simulink model "modelo_f_HIL"  (R2024b)
settings: Solver=ode15s  StartTime=0.0  StopTime=inf  FixedStep=T_s  RelTol=1e-3
InitFcn:
  | clc
  | clear
  | close all
  | clear all
  | clear mex
  | parametros
  | gain_CL
  | calculo_observador_carro
  | calculo_observador_izaje
values from neighbouring files (symbols this model uses):
  b_cx = 1e6    (= 1000000)    [parametros.m]
  b_cy = 1e7    (= 10000000)    [parametros.m]
  b_hb = 1e8    (= 100000000)    [parametros.m]
  b_hd = 8    [parametros.m]
  b_hm = 18    [parametros.m]
  b_t = 90    [parametros.m]
  b_tb = 5e6    (= 5000000)    [parametros.m]
  b_td = 1.8    [parametros.m]
  b_tm = 6    [parametros.m]
  b_tw = 3e3    (= 3000)    [parametros.m]
  b_wu = 150    [parametros.m]
  container_pillars = container_pillars(randperm(19))    [parametros.m]
  escenario = 1    [parametros.m]
  g = 9.80665    [parametros.m]
  H_c = 2.59    [parametros.m]
  H_truck = 1    [parametros.m]
  i_h = 22    [parametros.m]
  i_t = 30    [parametros.m]
  J_hd_hEb = 3800    [parametros.m]
  J_hm_hb = 30    [parametros.m]
  J_td = 1200    [parametros.m]
  J_tm_tb = 7    [parametros.m]
  K_cy = 1.8e9    (= 1800000000)    [parametros.m]
  K_tw = 4.8e5    (= 480000)    [parametros.m]
  k_wu = 2.36e8    (= 236000000)    [parametros.m]
  l_h0 = (Y_t0-y_l0)    (= 15)    [parametros.m]
  l_h_max = Y_t0-y_h_min    (= 65)    [parametros.m]
  l_h_maxE = l_h_max+0.5    (= 65.5)    [parametros.m]
  l_h_min = Y_t0-y_h_max    (= 5)    [parametros.m]
  l_h_minE = l_h_min-0.5    (= 4.5)    [parametros.m]
  M_cmax = 50000    [parametros.m]
  M_cmin = 2000    [parametros.m]
  M_s = 15000    [parametros.m]
  M_t = 30000    [parametros.m]
  r_hd = 0.75    [parametros.m]
  r_td = 0.50    (= 0.5)    [parametros.m]
  T_hbMax = 5e4    (= 50000)    [parametros.m]
  T_hEbMax = 1.1e6    (= 1100000)    [parametros.m]
  T_hmMax = 2e4    (= 20000)    [parametros.m]
  T_s = 0.001    [parametros.m]
  T_s0 = 0.001    [parametros.m]
  T_s1 = 0.020    (= 0.02)    [parametros.m]
  T_s2 = 0.020    (= 0.02)    [parametros.m]
  T_tbMax = 5e3    (= 5000)    [parametros.m]
  T_tmMax = 4e3    (= 4000)    [parametros.m]
  tau_tm = 1e-3    (= 0.001)    [parametros.m]
  theta_hm0 = -l_h0*i_h*2/r_hd    (= -880)    [parametros.m]
  theta_tm0 = (x_t0)*i_t/r_td    (= -1500)    [parametros.m]
  trucks0 = [0, 0, 0, 0, 0]    [parametros.m]
  v_h_max_load = 1.5    [parametros.m]
  v_h_max_noload = 3    [parametros.m]
  v_lx0 = 0    [parametros.m]
  v_ly0 = 0    [parametros.m]
  v_t0 = 0    [parametros.m]
  v_t_max = 4    [parametros.m]
  W_c = ctrb(A, B_c(:,1))    [CyO_carro.m]    (also in CyO_izaje.m; parametros.m = 2.44)
  w_hm0 = 0    [parametros.m]
  w_hm_rated = v_h_max_load*2*i_h/r_hd    (= 88)    [parametros.m]
  w_tm0 = (v_t0)*i_t/r_td    (= 0)    [parametros.m]
  x_c0_left = -35    [parametros.m]
  x_c0_right = 55    [parametros.m]
  x_containers_left_lim = 1.5    [parametros.m]
  x_containers_right_lim = 48.5    [parametros.m]
  x_l0 = x_t0    (= -25)    [parametros.m]
  x_lidar_offset = 3.0    (= 3)    [parametros.m]
  x_t0 = -25    [parametros.m]
  x_t_max = 50    [parametros.m]
  x_t_maxE = x_t_max+0.5    (= 50.5)    [parametros.m]
  x_t_min = -30    [parametros.m]
  x_t_minE = x_t_min-0.5    (= -30.5)    [parametros.m]
  y_h_min = -20    [parametros.m]
  y_l0 = 30    [parametros.m]
  Y_sb = 5.0    (= 5)    [parametros.m]
  Y_t0 = 45    [parametros.m]
libraries: opcualib x2, dspnetwork x2, dspsigops x1, simulink x1
(part 3 of 3)

== matlab function modelo_f_HIL/UDP: Controller reader/MATLAB Function ==
  data: trolley_cmd output; hoist_cmd output; system_on output; auto_mode output; twistlock output; sway_ctrl output; emergency output; emgy_ack output; data input
function [trolley_cmd, hoist_cmd, system_on, auto_mode, twistlock, sway_ctrl, emergency, emgy_ack] = parse_udp_packet(data)
% parse_udp_packet  Desempaqueta el datagrama de 14 bytes enviado por controller_reader.py
%
% Entrada:
%   data  : uint8(1x14) — bytes crudos del bloque UDP Receive
%
% Salidas (todas double):
%   trolley_cmd  [-4.0 .. +4.0] m/s   consigna velocidad carro
%   hoist_cmd    [-1.5 .. +1.5] m/s   consigna velocidad izaje
%   system_on    0/1   Sistema ON/OFF
%   auto_mode    0/1   Modo automático activo
%   twistlock    0/1   0=Abierto 1=Cerrado
%   sway_ctrl    0/1   Control de balanceo ON/OFF
%   emergency    0/1   Emergencia activa
%   emgy_ack     0/1   ACK de emergencia global
%
% Formato del paquete Python: struct.pack('!ffBBBBBB', ...)
%   Big-endian: bytes 1-4 float32, 5-8 float32, 9-14 uint8
% -----------------------------------------------------------------------

% Valores por defecto (paquete malformado o vacío)
trolley_cmd = 0;
hoist_cmd   = 0;
system_on   = 0;
auto_mode   = 0;
twistlock   = 0;
sway_ctrl   = 0;
emergency   = 0;
emgy_ack    = 0;

if numel(data) < 14
    return
end

raw = uint8(data(:)');   % forzar fila 1x14

% ── Floats big-endian → invertir bytes antes de typecast ──────────────
%    Python '!' = big-endian; x86/MATLAB = little-endian
trolley_cmd = double(typecast(raw(4:-1:1), 'single'));
hoist_cmd   = double(typecast(raw(8:-1:5), 'single'));

% ── Flags uint8 (un byte cada uno) ────────────────────────────────────
system_on = double(raw(9));
auto_mode = double(raw(10));
twistlock = double(raw(11));
sway_ctrl = double(raw(12));
emergency = double(raw(13));
emgy_ack  = double(raw(14));

== matlab function modelo_f_HIL/Nivel 2/MATLAB Function5 ==
  data: x_t_ref input; v_t_ref output; x_hat input; v_t_ff input; v_td_hat input; v_max input
function v_t_ref = controlador_posicion(x_t_ref, x_hat, v_t_ff,v_td_hat, v_max)

    % Kp = 2;
    Kd = 0;
    Kp = .11;

    e_x = x_t_ref - x_hat;
    % e_v = v_t_ff - v_td_hat;

    % v_calculada = (Kp * e_x) + e_v* Kd;
    v_calculada = Kp * e_x  + v_t_ff* Kd;

    if v_calculada > v_max
        v_t_ref = v_max;
    elseif v_calculada < -v_max
        v_t_ref = -v_max;
    else
        v_t_ref = v_calculada;
    end
end

== matlab function modelo_f_HIL/Nivel 2/MATLAB Function6 ==
  data: dl_h_ref output; l_h_ref input; l_h_sensor input; dl_h_ff input; m_est input
function dl_h_ref = controlador_posicion(l_h_ref, l_h_sensor, dl_h_ff, m_est)

    Kp = 0.5;

    e_l_h = l_h_ref - l_h_sensor;

    dl_h_ref = Kp * e_l_h; %+ dl_h_ff;

    if m_est > 16000
        dl_h_ref = min([1.5, max([dl_h_ref, -1.5])]);
    else
        dl_h_ref = min([3, max([dl_h_ref, -3])]);
    end
end

== matlab function modelo_f_HIL/Nivel 2/MATLAB Function2 ==
  data: sway_ctr_gain input; theta_hm input; theta_l input; v_balanceo output; w_l input; w_hm_hat input; enable input
function v_balanceo = controlador_balanceo_torque(sway_ctr_gain, theta_hm, theta_l, w_l, w_hm_hat, enable)
    persistent g r_hd i_h DEG2RAD 

    if isempty(g)
        DEG2RAD = pi/180;
        g       = 9.8066;
        r_hd    = 0.75;
        i_h     = 22;
    end

    if ~enable
        v_balanceo = 0;
        return;
    end

    l      = theta_hm * (-r_hd)/(i_h*2);
    dl_dt  = w_hm_hat * (-r_hd)/(i_h*2);
    l_seg  = max(l, 0.1);
    th_sat = max(-80*DEG2RAD, min(80*DEG2RAD, theta_l));
    w_o    = sqrt(g / l_seg);
    K_do   = (2*w_o*l_seg - 2*dl_dt) / cos(th_sat);
    v_balanceo = K_do * theta_l;   

end

== matlab function modelo_f_HIL/Nivel 2/Subsistema físico/MATLAB Function ==
  data: x_c0_left input; y_c0_contacto output; x_c0_right input; Y_sb input; W_c input; y_h_min input; H_c input; x_lidar_offset input; x_l input; container_pillars input; TLK input; x_t input; trucks0 input; H_truck input; Ts input; rand_in input; escenario input; x_containers_left_lim input; x_containers_right_lim input; t_camion_transicion input; y_c0_lidar output; containers_pillars_state output size=1,19; trucks_state output; trucks_has_load output; carga_tomada output
function [y_c0_contacto, y_c0_lidar, containers_pillars_state, trucks_state, trucks_has_load, carga_tomada] = ...
    perfil_suelo(x_c0_left, x_c0_right, Y_sb, W_c, y_h_min, H_c, x_lidar_offset, x_l, ...
                 container_pillars, TLK, x_t, trucks0, H_truck, Ts, rand_in, escenario, ...
                 x_containers_left_lim, x_containers_right_lim, t_camion_transicion)

persistent n_containers x_grid2 tlk_prev dx_grid idx_posiciones
persistent trucks_state_p trucks_has_load_p idx_trucks lambda_truck grupo_camion
persistent idx_zona_min idx_zona_max
persistent truck_en_transicion truck_timer
persistent carga_tomada_p

% Declarar tamaño variable seguro para arreglos dinámicos persistentes
coder.varsize('x_grid2', [1, 10000], [false, true]);
coder.varsize('n_containers', [1, 10000], [false, true]);

%% Inicialización de perfil de contenedores
if isempty(n_containers)
    dx_grid = 0.01;
    x_grid2 = x_c0_left : dx_grid : x_c0_right;
    n_containers = zeros(1, length(x_grid2));
    tlk_prev     = false;
    
    % --- Limites de la zona valida de contenedores (nunca escribir fuera de esto) ---
    idx_zona_min = round((x_containers_left_lim - x_c0_left) / dx_grid) + 1;
    idx_zona_max = round((x_containers_right_lim - x_c0_left) / dx_grid) + 1;
    idx_zona_min = max(1, min(length(x_grid2), idx_zona_min));
    idx_zona_max = max(1, min(length(x_grid2), idx_zona_max));
    
    % --- Carga inicial de pilas (19 posiciones estáticas garantizadas 1x19) ---
    n_pilares = 19;
    x_posiciones = linspace(x_containers_left_lim, x_containers_right_lim, n_pilares);
    idx_posiciones = zeros(1, 19);
    medio_ancho_idx = round((W_c/2) / dx_grid);
    
    for k = 1:n_pilares
        idx_pos = round((x_posiciones(k) - x_c0_left) / dx_grid) + 1;
        idx_pos = max(1, min(length(x_grid2), idx_pos));
        idx_posiciones(k) = idx_pos;
        
        idx_ini = max([1, idx_pos - medio_ancho_idx, idx_zona_min]);
        idx_fin = min([length(x_grid2), idx_pos + medio_ancho_idx, idx_zona_max]);
        n_containers(idx_ini:idx_fin) = container_pillars(k);
    end
    
    % --- Inicialización de camiones ---
    x_trucks_left = [-25 -20 -15 -10 -5];
    idx_trucks = zeros(1, 5);
    for k = 1:5
        idx_t = round((x_trucks_left(k) - x_c0_left) / dx_grid) + 1;
        idx_trucks(k) = max(1, min(length(x_grid2), idx_t));
    end
    
    trucks_state_p      = double(trucks0(:)'); % Forzar dimensiones 1x5
    trucks_has_load_p   = zeros(1,5);
    lambda_truck        = -log(0.5) / 60;
    grupo_camion        = ones(1,5);
    truck_en_transicion = zeros(1,5);
    truck_timer         = zeros(1,5);
    carga_tomada_p      = false;
end

%% Índice más cercano a x_l (posición de la carga)
idx = round((x_l - x_c0_left) / dx_grid) + 1;
idx = max(1, min(length(x_grid2), idx));
medio_ancho_idx = round((W_c/2) / dx_grid);

% La ventana de escritura/lectura de la carga nunca invade fuera
% de la zona valida de contenedores (evita que se mezcle con Y_sb u otras zonas)
idx_ini_l = max([1, idx - medio_ancho_idx, idx_zona_min]);
idx_fin_l = min([length(x_grid2), idx + medio_ancho_idx, idx_zona_max]);

%% Flancos de TLK
tlk_bool      = logical(TLK);
flanco_bajada = tlk_prev && ~tlk_bool;   % Soltar carga (1 -> 0)
flanco_subida = ~tlk_prev && tlk_bool;   % Tomar carga (0 -> 1)
tlk_prev      = tlk_bool;

% carga_tomada refleja directamente si el spreader esta enganchado a algo
% (TLK activo).
if flanco_subida
    carga_tomada_p = true;
elseif flanco_bajada
    carga_tomada_p = false;
end
carga_tomada = carga_tomada_p;

%% Identificar si la carga está sobre la posición de un camión
W_trucks_idx = round((W_c/2) / dx_grid);
sobre_camion_k = 0;
for k = 1:5
    if abs(idx - idx_trucks(k)) <= W_trucks_idx && trucks_state_p(k) == 1
        sobre_camion_k = k;
        break;
    end
end

%% Manejo de escenarios
if escenario ~= 0
    switch escenario
        case 1
            grupo_camion = ones(1,5);     % Carga
        case 2
            grupo_camion = 2*ones(1,5);   % Descarga
        case 3
            grupo_camion = [2 2 1 1 1];   % Mixto
    end
end

if sobre_camion_k > 0 && escenario ~= 0
    k = sobre_camion_k;
    if flanco_subida && grupo_camion(k) == 1 && trucks_has_load_p(k) == 1
        % El camión libera la carga instantáneamente al spreader
        trucks_has_load_p(k) = 0; 
        
        % Se arma un timer. El camión VACÍO se retira recién después
        truck_en_transicion(k) = 1;
        truck_timer(k) = 0;
        
    elseif flanco_bajada && grupo_camion(k) == 2 && trucks_has_load_p(k) == 0
        % NUEVA CORRECCIÓN: Al depositar, el camión recibe la carga instantáneamente
        trucks_has_load_p(k) = 1; 
        
        % Inicia el timer. El camión (CON CARGA) se retirará después de t_camion_transicion
        truck_en_transicion(k) = 1;
        truck_timer(k) = 0;
    end
else
    % Solo modifica n_containers si la ventana de escritura cae dentro de la zona valida
    if idx_fin_l >= idx_ini_l
        
        % Buscar el pilar fijo más cercano a la posición de la carga
        [dist_min, pilar_cercano] = min(abs(idx - idx_posiciones));
        
        % Si la carga está sobre uno de los pilares del barco/patio (tolerancia de medio ancho)
        if dist_min <= medio_ancho_idx
            % Hacemos "snap" a los índices exactos con los que se inicializó ese pilar
            idx_centro = idx_posiciones(pilar_cercano);
            idx_ini_write = max([1, idx_centro - medio_ancho_idx, idx_zona_min]);
            idx_fin_write = min([length(x_grid2), idx_centro + medio_ancho_idx, idx_zona_max]);
        else
            % Si está depositando fuera de las zonas predefinidas (caída libre)
            idx_ini_write = idx_ini_l;
            idx_fin_write = idx_fin_l;
        end
        
        if flanco_bajada
            altura_actual = max(n_containers(idx_ini_write:idx_fin_write));
            n_containers(idx_ini_write:idx_fin_write) = max(n_containers(idx_ini_write:idx_fin_write), altura_actual + 1);
        elseif flanco_subida
            altura_actual = max(n_containers(idx_ini_write:idx_fin_write));
            n_containers(idx_ini_write:idx_fin_write) = max(0, altura_actual - 1);
        end
    end
end

%% Reaparición probabilística
if escenario ~= 0
    p_ciclo = 1 - exp(-lambda_truck * Ts);
    for k = 1:5
        if trucks_state_p(k) == 0
            if rand_in(k) < p_ciclo
                trucks_state_p(k) = 1;
                if grupo_camion(k) == 1
                    trucks_has_load_p(k) = 1;
                else
                    trucks_has_load_p(k) = 0;
                end
                truck_en_transicion(k) = 0; % camion nuevo, sin transicion pendiente
                truck_timer(k) = 0;
            end
        end
    end
end

%% Altura fija según zona
if x_l < -1
    y_fijo = 0;
elseif x_l >= -1 && x_l <= 0
    y_fijo = Y_sb;
else
    y_fijo = y_h_min;
end

%% Aporte de altura de camiones
h_truck_l = 0;
for k = 1:5
    if abs(idx - idx_trucks(k)) <= W_trucks_idx && trucks_state_p(k) == 1
        % Discriminar entre camión con carga y plataforma vacía
        if trucks_has_load_p(k) == 1
            h_truck_l = H_truck + H_c; % Altura con contenedor (activo durante los 30s de salida)
        else
            h_truck_l = H_truck;       % Altura solo de la plataforma
        end
    end
end

%% Altura total de contacto
if idx_fin_l >= idx_ini_l
    altura_containers_l = max(n_containers(idx_ini_l:idx_fin_l));
else
    altura_containers_l = 0;
end
y_c0_contacto = y_fijo + altura_containers_l * H_c + h_truck_l;

%% Resolucion de camiones en transicion (basado en TIEMPO)
% Cada camion en transicion incrementa su timer en cada paso; cuando
% supera t_camion_transicion segundos, recien ahi desaparece de verdad.
for k = 1:5
    if truck_en_transicion(k) == 1
        truck_timer(k) = truck_timer(k) + Ts;
        if truck_timer(k) >= t_camion_transicion
            trucks_state_p(k)      = 0;
            trucks_has_load_p(k)   = 0; % Limpia el camión y su carga
            truck_en_transicion(k) = 0;
            truck_timer(k)         = 0;
        end
    end
end

%% Lectura de Lidar
x_laser = x_t + x_lidar_offset;
idx_lidar = round((x_laser - x_c0_left) / dx_grid) + 1;
idx_lidar = max(1, min(length(x_grid2), idx_lidar));

if x_laser < -1
    y_fijo_lidar = 0;
elseif x_laser >= -1 && x_laser <= 0
    y_fijo_lidar = Y_sb;
else
    y_fijo_lidar = y_h_min;
end

h_truck_lidar = 0;
for k = 1:5
    if abs(idx_lidar - idx_trucks(k)) <= W_trucks_idx && trucks_state_p(k) == 1
        if trucks_has_load_p(k) == 1
            h_truck_lidar = H_truck + H_c;
        else
            h_truck_lidar = H_truck;
        end
    end
end
y_c0_lidar = y_fijo_lidar + n_containers(idx_lidar) * H_c + h_truck_lidar;

%% Salidas garantizadas
containers_pillars_state = n_containers(idx_posiciones);
trucks_state              = trucks_state_p;
trucks_has_load           = trucks_has_load_p;
end

== matlab function modelo_f_HIL/Nivel 2/MATLAB Function ==
  data: v_t_star input; T_tm_star output; v_td_hat input
function T_tm_star = PID_carro(v_t_star, v_td_hat)

    persistent int1 int2 k_tsia k_tsa b_ta T_s e_prev int1_prev e_x_t_prev;

    if isempty(int1)
        int1 = 0;
        int2 = 0;
        k_tsia = 817.1486;
        k_tsa = 4.09*10^3;
        b_ta = 4.3394*10^3;
        T_s = 0.001;
        e_prev = 0;
        int1_prev = 0;
        e_x_t_prev = 0;
    end

    e_t = v_t_star - v_td_hat;

    int1 = int1 + T_s * (e_t+e_prev)/2;
    e_prev = e_t;
    int2 = int2 + T_s * (int1+int1_prev)/2;
    int1_prev = int1;



    T_tm_star = e_t * b_ta + (int1) * k_tsa + int2 * k_tsia;

end

== matlab function modelo_f_HIL/Nivel 2/MATLAB Function1 ==
  data: F_hw input; T_hm_star output; dl_h_star input; w_hm_hat input
function T_hm_star = fcn(F_hw, dl_h_star, w_hm_hat)

persistent int1 int2 k_hsia k_hsa b_ha T_s r_hd i_h e_prev int1_prev

if isempty(int1)

    int1 = 0;
    int2 = 0;
    k_hsia = -6.4992*10^5;
    k_hsa = -4.3987*10^5;
    b_ha = -6.7646*10^4;
    T_s = 0.001;
    r_hd = 0.75;
    i_h = 22;
    e_prev = 0;
    int1_prev = 0;

end

dl_h = w_hm_hat * (-r_hd)/(i_h*2);

e_h = dl_h_star - dl_h;

int1 = int1 + T_s * (e_h+e_prev)/2;

e_prev = e_h;

int2 = int2 + T_s * (int1+int1_prev)/2;

int1_prev = int1;

T_hm_star = F_hw*r_hd/(i_h*2) + b_ha * e_h + k_hsa * int1 + k_hsia * int2;

end

== matlab function modelo_f_HIL/Nivel 2/MATLAB Function3 ==
  data: theta_tm input; out_theta_tm_hat output; F_hw input; theta_l input; T_tm input; out_omega_tm_hat output; out_x_t_hat output; out_v_t_hat output
function [out_theta_tm_hat, out_omega_tm_hat, out_x_t_hat, out_v_t_hat] = fcn(theta_tm, F_hw, theta_l, T_tm)

persistent r_td i_t K_tw b_tw b_t M_t T_s Lt1 Lt2 Lt3 Lt4 J_tEq b_tEq dv_t_hat_prev v_t_hat_prev w_tm_hat_prev dw_tm_hat_prev w_tm_hat theta_tm_hat dw_tm_hat x_t_hat v_t_hat
 
if isempty(r_td)

    r_td = 0.5;
    i_t = 30;
    K_tw = 480000;
    b_tw = 3000;
    b_t = 90;
    M_t = 30000;
    T_s = 0.001;
    Lt1 = 11.0536;
    Lt2 = 11.5001;
    Lt3 = -0.0851;
    Lt4 = -0.2405;
    J_tEq = 8.3333;
    b_tEq = 6.06;
    dv_t_hat_prev = 0;
    v_t_hat_prev = 0;
    x_t_hat = theta_tm*r_td/i_t;
    v_t_hat = 0;
    theta_tm_hat = theta_tm;
    dw_tm_hat_prev = 0;
    w_tm_hat = 0;
    w_tm_hat_prev = 0;
   
end

    e_theta = theta_tm - theta_tm_hat;

    F_tw = (theta_tm*(r_td/i_t) - x_t_hat)*K_tw + (w_tm_hat*(r_td/i_t) - v_t_hat) * b_tw;

    dv_t_hat = (1/M_t) * (2*F_hw*sin(theta_l) - b_t*v_t_hat + F_tw) + Lt4 * e_theta;
    v_t_hat = v_t_hat + T_s * (dv_t_hat+dv_t_hat_prev)/2 + Lt3 * e_theta;
    dv_t_hat_prev = dv_t_hat;
    x_t_hat = x_t_hat + T_s * (v_t_hat+v_t_hat_prev)/2;
    v_t_hat_prev = v_t_hat;
 
    dw_tm_hat = (1/J_tEq)*(T_tm - F_tw*(r_td/i_t)) - w_tm_hat * b_tEq + Lt2 * e_theta;
    w_tm_hat = w_tm_hat + T_s * (dw_tm_hat_prev+dw_tm_hat)/2 + Lt1 * e_theta;
    dw_tm_hat_prev = dw_tm_hat;
    theta_tm_hat = theta_tm_hat + T_s * (w_tm_hat+w_tm_hat_prev)/2;
    w_tm_hat_prev = w_tm_hat;

    out_theta_tm_hat = theta_tm_hat;
    out_omega_tm_hat = w_tm_hat;
    out_x_t_hat      = x_t_hat;
    out_v_t_hat      = v_t_hat;
    
end
